simulink library "slexPowerWindowSALib"  (R2014b)
settings: Solver=ode45  SolverMode=SingleTasking  StartTime=0.0  StopTime=10.0  RelTol=1e-3
libraries: slexPowerWindowSALib x4, simulink x2
Description:
  | Library of Components for Control System
settings Model: ExtModeAutoUpdateStatusClock=off  Creator=The MathWorks Inc.  LastModifiedBy=The MathWorks Inc.

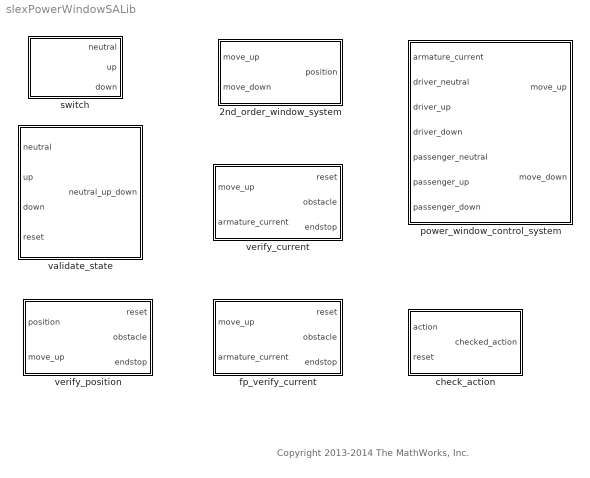
== system slexPowerWindowSALib ==
  note: Copyright 2013-2014 The MathWorks, Inc.
  2nd_order_window_system : Subsystem
  check_action : Subsystem
  fp_verify_current : Subsystem
  power_window_control_system : Subsystem
  switch : Subsystem
  validate_state : Subsystem
  verify_current : Subsystem
  verify_position : Subsystem

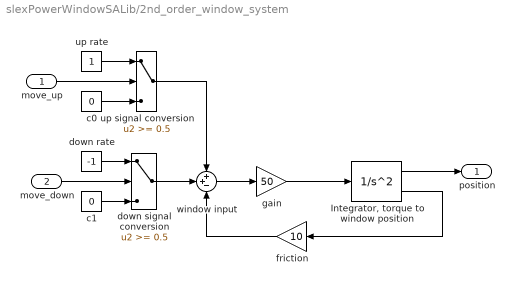
== system slexPowerWindowSALib/2nd_order_window_system ==
  move_up : Inport
  move_down : Inport  Port=2
  "Integrator, torque to window position " : SecondOrderIntegrator
  c0 : Constant  Value=0
  c1 : Constant  Value=0
  down rate : Constant  Value=-1
  down signal conversion : Switch  Threshold=0.5  SaturateOnIntegerOverflow=on  InputSameDT=on
  friction : Gain  Gain=10  SaturateOnIntegerOverflow=on  OutDataTypeStr=Inherit: Same as input  ParamDataTypeStr=Inherit: Same as input
  gain : Gain  Gain=50  SaturateOnIntegerOverflow=on  OutDataTypeStr=Inherit: Same as input  ParamDataTypeStr=Inherit: Same as input
  up rate : Constant
  up signal conversion : Switch  Threshold=0.5  SaturateOnIntegerOverflow=on  InputSameDT=on
  window input : Sum  Inputs=++-  SaturateOnIntegerOverflow=on  InputSameDT=on  OutDataTypeStr=Inherit: Same as first input
  position : Outport
  wires:
  move_down/1 -> down signal conversion/2
  "Integrator, torque to window position "/1 -> position/1
  move_up/1 -> up signal conversion/2
  up rate/1 -> up signal conversion/1
  c0/1 -> up signal conversion/3
  down rate/1 -> down signal conversion/1
  c1/1 -> down signal conversion/3
  up signal conversion/1 -> window input/1
  down signal conversion/1 -> window input/2
  window input/1 -> gain/1
  gain/1 -> "Integrator, torque to window position "/1
  "Integrator, torque to window position "/2 -> friction/1
  friction/1 -> window input/3

== system slexPowerWindowSALib/check_action ==
  action : Inport
  reset : Inport  Port=2
  allow_action : Logic  IconShape=distinctive  OutDataTypeStr=boolean
  overrule : Logic  Operator=NOT  IconShape=distinctive  OutDataTypeStr=boolean
  checked_action : Outport
  wires:
  overrule/1 -> allow_action/2
  action/1 -> allow_action/1
  allow_action/1 -> checked_action/1
  reset/1 -> overrule/1

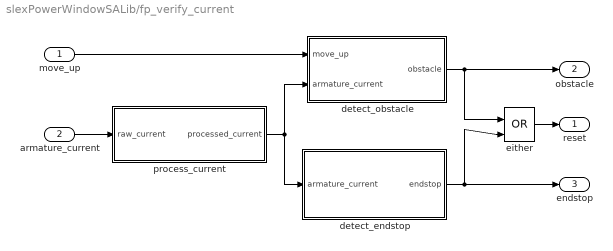
== system slexPowerWindowSALib/fp_verify_current ==
  move_up : Inport  OutDataTypeStr=boolean
  armature_current : Inport  Port=2
  detect_endstop : Subsystem
  detect_obstacle : Subsystem
  either : Logic  Operator=OR  IconShape=distinctive  OutDataTypeStr=boolean
  process_current : Subsystem
  reset : Outport
  obstacle : Outport  Port=2
  endstop : Outport  Port=3
  wires:
  armature_current/1 -> process_current/1(raw_current)
  detect_obstacle/1(obstacle) -> either/1, obstacle/1
  detect_endstop/1(endstop) -> endstop/1, either/2
  either/1 -> reset/1
  move_up/1 -> detect_obstacle/1(move_up)
  process_current/1(processed_current) -> detect_obstacle/2(armature_current), detect_endstop/1(armature_current)

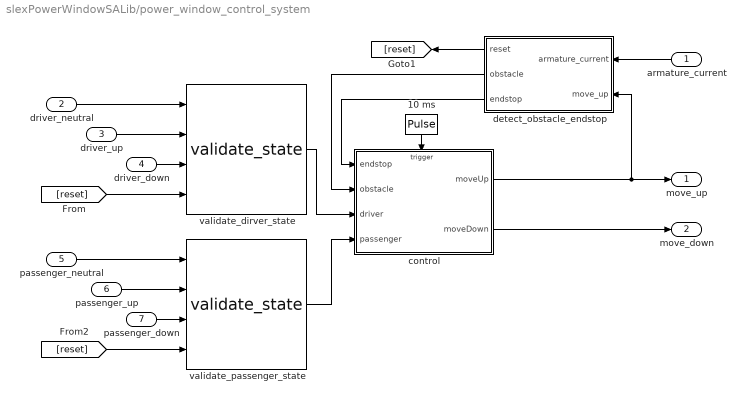
== system slexPowerWindowSALib/power_window_control_system ==
  armature_current : Inport
  driver_neutral : Inport  Port=2
  driver_up : Inport  Port=3
  driver_down : Inport  Port=4
  passenger_neutral : Inport  Port=5
  passenger_up : Inport  Port=6
  passenger_down : Inport  Port=7
  10 ms : DiscretePulseGenerator  PulseType=Time based  Period=1e-2  SampleTime=1e-3
  control : Stateflow chart  TreatAsAtomicUnit=on
  detect_obstacle_endstop : Subsystem
  validate_dirver_state : slexPowerWindowSALib/validate_state
  validate_passenger_state : slexPowerWindowSALib/validate_state
  move_up : Outport
  move_down : Outport  Port=2
  wires:
  armature_current/1 -> detect_obstacle_endstop/1(armature_current)
  control/2(moveDown) -> move_down/1
  control/1(moveUp) -> detect_obstacle_endstop/2(move_up), move_up/1
  detect_obstacle_endstop/3(endstop) -> control/1(endstop)
  detect_obstacle_endstop/2(obstacle) -> control/2(obstacle)
  validate_passenger_state/1 -> control/4(passenger)
  validate_dirver_state/1 -> control/3(driver)
  10 ms/1 -> control/Trigger
  detect_obstacle_endstop/1(reset) -> [reset]
  [reset] -> validate_passenger_state/4
  passenger_down/1 -> validate_passenger_state/3
  passenger_up/1 -> validate_passenger_state/2
  passenger_neutral/1 -> validate_passenger_state/1
  driver_down/1 -> validate_dirver_state/3
  driver_up/1 -> validate_dirver_state/2
  driver_neutral/1 -> validate_dirver_state/1
  [reset] -> validate_dirver_state/4

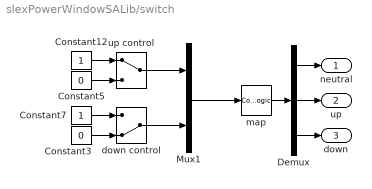
== system slexPowerWindowSALib/switch ==
  Constant12 : Constant  OutDataTypeStr=boolean
  Constant3 : Constant  Value=0  OutDataTypeStr=boolean
  Constant5 : Constant  Value=0  OutDataTypeStr=boolean
  Constant7 : Constant  OutDataTypeStr=boolean
  Demux : Demux  Outputs=3
  Mux1 : Mux  Inputs=2
  down control : ManualSwitch  CurrentSetting=0
  map : CombinatorialLogic  TruthTable=[1 0 0;0 0 1;0 1 0;1 0 0]
  up control : ManualSwitch
  neutral : Outport
  up : Outport  Port=2
  down : Outport  Port=3
  wires:
  Demux/3 -> down/1
  Demux/2 -> up/1
  Demux/1 -> neutral/1
  map/1 -> Demux/1
  up control/1 -> Mux1/1
  down control/1 -> Mux1/2
  Constant3/1 -> down control/2
  Constant7/1 -> down control/1
  Constant5/1 -> up control/2
  Constant12/1 -> up control/1
  Mux1/1 -> map/1

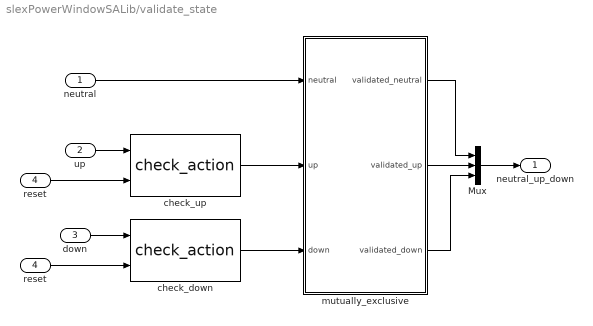
== system slexPowerWindowSALib/validate_state ==
  neutral : Inport
  up : Inport  Port=2
  down : Inport  Port=3
  reset : Inport  Port=4
  Mux : Mux  Inputs=3
  check_down : slexPowerWindowSALib/check_action
  check_up : slexPowerWindowSALib/check_action
  mutually_exclusive : Subsystem
  "reset " : InportShadow  Port=4
  neutral_up_down : Outport
  wires:
  check_down/1 -> mutually_exclusive/3(down)
  mutually_exclusive/3(validated_down) -> Mux/3
  mutually_exclusive/2(validated_up) -> Mux/2
  mutually_exclusive/1(validated_neutral) -> Mux/1
  down/1 -> check_down/1
  up/1 -> check_up/1
  neutral/1 -> mutually_exclusive/1(neutral)
  check_up/1 -> mutually_exclusive/2(up)
  "reset "/1 -> check_up/2
  reset/1 -> check_down/2
  Mux/1 -> neutral_up_down/1

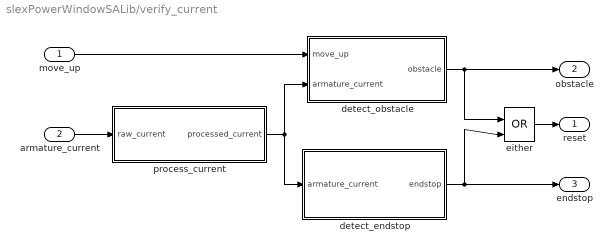
== system slexPowerWindowSALib/verify_current ==
  move_up : Inport  OutDataTypeStr=boolean
  armature_current : Inport  Port=2
  detect_endstop : Subsystem
  detect_obstacle : Subsystem
  either : Logic  Operator=OR  IconShape=distinctive  OutDataTypeStr=boolean
  process_current : Subsystem
  reset : Outport
  obstacle : Outport  Port=2
  endstop : Outport  Port=3
  wires:
  process_current/1(processed_current) -> detect_endstop/1(armature_current), detect_obstacle/2(armature_current)
  move_up/1 -> detect_obstacle/1(move_up)
  either/1 -> reset/1
  detect_endstop/1(endstop) -> either/2, endstop/1
  detect_obstacle/1(obstacle) -> obstacle/1, either/1
  armature_current/1 -> process_current/1(raw_current)

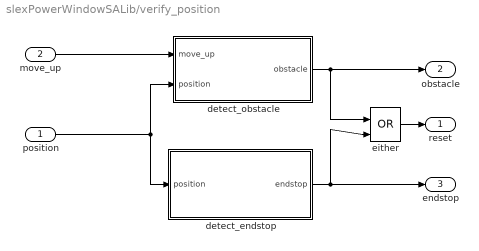
== system slexPowerWindowSALib/verify_position ==
  position : Inport
  move_up : Inport  Port=2  OutDataTypeStr=boolean
  detect_endstop : Subsystem
  detect_obstacle : Subsystem
  either : Logic  Operator=OR  IconShape=distinctive  OutDataTypeStr=boolean
  reset : Outport
  obstacle : Outport  Port=2
  endstop : Outport  Port=3
  wires:
  move_up/1 -> detect_obstacle/1(move_up)
  position/1 -> detect_endstop/1(position), detect_obstacle/2(position)
  either/1 -> reset/1
  detect_endstop/1(endstop) -> either/2, endstop/1
  detect_obstacle/1(obstacle) -> obstacle/1, either/1

== system slexPowerWindowSALib/fp_verify_current/detect_endstop ==
  armature_current : Inport
  current_limit : simulink/Logic and Bit Operations/Compare To Constant  relop=>  const=15  OutDataTypeStr=boolean
  endstop : Outport
  wires:
  current_limit/1 -> endstop/1
  armature_current/1 -> current_limit/1

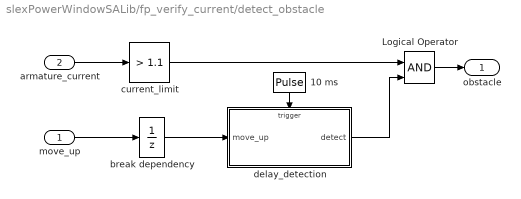
== system slexPowerWindowSALib/fp_verify_current/detect_obstacle ==
  move_up : Inport  OutDataTypeStr=boolean
  armature_current : Inport  Port=2
  10 ms : DiscretePulseGenerator  SampleTime=10e-3
  Logical Operator : Logic  IconShape=distinctive  AllPortsSameDT=off  OutDataTypeStr=boolean
  break dependency : UnitDelay  SampleTime=0.01
  current_limit : simulink/Logic and Bit Operations/Compare To Constant  relop=>  const=1.1  OutDataTypeStr=boolean
  delay_detection : Stateflow chart  TreatAsAtomicUnit=on
  obstacle : Outport
  wires:
  break dependency/1 -> delay_detection/1(move_up)
  10 ms/1 -> delay_detection/Trigger
  move_up/1 -> break dependency/1
  armature_current/1 -> current_limit/1
  delay_detection/1(" detect") -> Logical Operator/2
  current_limit/1 -> Logical Operator/1
  Logical Operator/1 -> obstacle/1

== system slexPowerWindowSALib/fp_verify_current/process_current ==
  raw_current : Inport
  3.5 / (2^(bits-1)) : Gain  Gain=0.02734375  OutDataTypeStr=fixdt(1,16,6)
  Abs : Abs
  gain : Gain  Gain=5  OutDataTypeStr=fixdt(1,16,5)
  processed_current : Outport
  wires:
  raw_current/1 -> 3.5 / (2^(bits-1))/1
  Abs/1 -> processed_current/1
  gain/1 -> Abs/1
  3.5 / (2^(bits-1))/1 -> gain/1

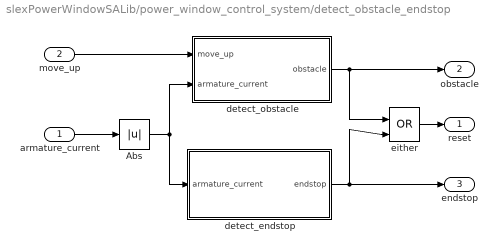
== system slexPowerWindowSALib/power_window_control_system/detect_obstacle_endstop ==
  armature_current : Inport
  move_up : Inport  Port=2
  Abs : Abs  SaturateOnIntegerOverflow=on
  detect_endstop : Subsystem
  detect_obstacle : Subsystem
  either : Logic  Operator=OR  IconShape=distinctive  OutDataTypeStr=boolean
  reset : Outport
  obstacle : Outport  Port=2
  endstop : Outport  Port=3
  wires:
  detect_obstacle/1(obstacle) -> either/1, obstacle/1
  detect_endstop/1(endstop) -> endstop/1, either/2
  either/1 -> reset/1
  armature_current/1 -> Abs/1
  move_up/1 -> detect_obstacle/1(move_up)
  Abs/1 -> detect_endstop/1(armature_current), detect_obstacle/2(armature_current)

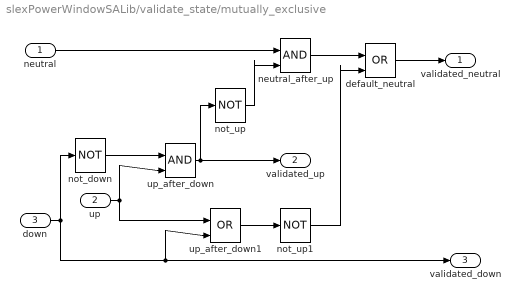
== system slexPowerWindowSALib/validate_state/mutually_exclusive ==
  neutral : Inport
  up : Inport  Port=2
  down : Inport  Port=3
  default_neutral : Logic  Operator=OR  IconShape=distinctive  OutDataTypeStr=boolean
  neutral_after_up : Logic  IconShape=distinctive  OutDataTypeStr=boolean
  not_down : Logic  Operator=NOT  IconShape=distinctive  OutDataTypeStr=boolean
  not_up : Logic  Operator=NOT  IconShape=distinctive  OutDataTypeStr=boolean
  not_up1 : Logic  Operator=NOT  IconShape=distinctive  OutDataTypeStr=boolean
  up_after_down : Logic  IconShape=distinctive  OutDataTypeStr=boolean
  up_after_down1 : Logic  Operator=OR  IconShape=distinctive  OutDataTypeStr=boolean
  validated_neutral : Outport
  validated_up : Outport  Port=2
  validated_down : Outport  Port=3
  wires:
  not_up1/1 -> default_neutral/2
  default_neutral/1 -> validated_neutral/1
  neutral_after_up/1 -> default_neutral/1
  up_after_down1/1 -> not_up1/1
  up/1 -> up_after_down/2, up_after_down1/1
  neutral/1 -> neutral_after_up/1
  down/1 -> validated_down/1, up_after_down1/2, not_down/1
  not_up/1 -> neutral_after_up/2
  up_after_down/1 -> validated_up/1, not_up/1
  not_down/1 -> up_after_down/1

== system slexPowerWindowSALib/verify_current/detect_endstop ==
  armature_current : Inport
  Constant6 : Constant  Value=15
  current_limit : RelationalOperator  Operator=>  OutDataTypeStr=boolean  InputSameDT=on
  endstop : Outport
  wires:
  Constant6/1 -> current_limit/2
  armature_current/1 -> current_limit/1
  current_limit/1 -> endstop/1

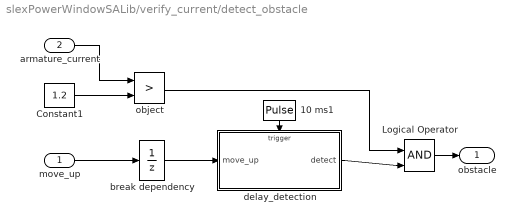
== system slexPowerWindowSALib/verify_current/detect_obstacle ==
  move_up : Inport  OutDataTypeStr=boolean
  armature_current : Inport  Port=2
  10 ms1 : DiscretePulseGenerator  SampleTime=10e-3
  Constant1 : Constant  Value=1.2
  Logical Operator : Logic  IconShape=distinctive  AllPortsSameDT=off  OutDataTypeStr=boolean
  break dependency : UnitDelay  SampleTime=0.01
  delay_detection : Stateflow chart  TreatAsAtomicUnit=on
  object : RelationalOperator  Operator=>  OutDataTypeStr=boolean  InputSameDT=on
  obstacle : Outport
  wires:
  Constant1/1 -> object/2
  object/1 -> Logical Operator/1
  delay_detection/1(" detect") -> Logical Operator/2
  armature_current/1 -> object/1
  move_up/1 -> break dependency/1
  10 ms1/1 -> delay_detection/Trigger
  break dependency/1 -> delay_detection/1(move_up)
  Logical Operator/1 -> obstacle/1

== system slexPowerWindowSALib/verify_current/process_current ==
  raw_current : Inport
  Abs : Abs  SaturateOnIntegerOverflow=on
  processed_current : Outport
  wires:
  Abs/1 -> processed_current/1
  raw_current/1 -> Abs/1

== system slexPowerWindowSALib/verify_position/detect_endstop ==
  position : Inport
  Constant1 : Constant  Value=0
  Constant6 : Constant  Value=0.4
  Logical Operator : Logic  Operator=OR  IconShape=distinctive  AllPortsSameDT=off  OutDataTypeStr=boolean
  bottom_limit : RelationalOperator  Operator=<  OutDataTypeStr=boolean  InputSameDT=on
  top_limit : RelationalOperator  Operator=>  OutDataTypeStr=boolean  InputSameDT=on
  endstop : Outport
  wires:
  Constant6/1 -> top_limit/2
  position/1 -> bottom_limit/1, top_limit/1
  Constant1/1 -> bottom_limit/2
  top_limit/1 -> Logical Operator/1
  bottom_limit/1 -> Logical Operator/2
  Logical Operator/1 -> endstop/1

== system slexPowerWindowSALib/verify_position/detect_obstacle ==
  move_up : Inport  OutDataTypeStr=boolean
  position : Inport  Port=2
  Break Dependency : Memory
  Constant1 : Constant  Value=0.3
  Logical Operator : Logic  IconShape=distinctive  AllPortsSameDT=off  OutDataTypeStr=boolean
  object : RelationalOperator  Operator=>  OutDataTypeStr=boolean  InputSameDT=on
  obstacle : Outport
  wires:
  Constant1/1 -> object/2
  object/1 -> Logical Operator/1
  position/1 -> object/1
  move_up/1 -> Break Dependency/1
  Break Dependency/1 -> Logical Operator/2
  Logical Operator/1 -> obstacle/1

== system slexPowerWindowSALib/power_window_control_system/detect_obstacle_endstop/detect_endstop ==
  armature_current : Inport
  Constant6 : Constant  Value=15
  current_limit : RelationalOperator  Operator=>  OutDataTypeStr=boolean  InputSameDT=on
  endstop : Outport
  wires:
  current_limit/1 -> endstop/1
  armature_current/1 -> current_limit/1
  Constant6/1 -> current_limit/2

== system slexPowerWindowSALib/power_window_control_system/detect_obstacle_endstop/detect_obstacle ==
  move_up : Inport
  armature_current : Inport  Port=2
  Constant1 : Constant  Value=1.6
  Logical Operator : Logic  IconShape=distinctive  AllPortsSameDT=off  OutDataTypeStr=boolean
  break dependency : UnitDelay  SampleTime=0.01
  delay 500 ms : Subsystem  TreatAsAtomicUnit=on
  object : RelationalOperator  Operator=>  OutDataTypeStr=boolean  InputSameDT=on
  obstacle : Outport
  wires:
  break dependency/1 -> delay 500 ms/Enable
  Logical Operator/1 -> obstacle/1
  move_up/1 -> break dependency/1
  armature_current/1 -> object/1
  delay 500 ms/1(step) -> Logical Operator/2
  object/1 -> Logical Operator/1
  Constant1/1 -> object/2

== system slexPowerWindowSALib/power_window_control_system/detect_obstacle_endstop/detect_obstacle/delay 500 ms ==
  Enable : EnablePort  StatesWhenEnabling=reset
  Constant : Constant
  Constant1 : Constant  Value=0.5
  Integrator : Integrator
  Relational Operator : RelationalOperator  Operator=>  OutDataTypeStr=boolean  InputSameDT=on
  step : Outport  OutputWhenDisabled=reset  InitialOutput=0
  wires:
  Relational Operator/1 -> step/1
  Constant1/1 -> Relational Operator/2
  Integrator/1 -> Relational Operator/1
  Constant/1 -> Integrator/1

== stateflow chart slexPowerWindowSALib/power_window_control_system/control ==
  settings: executeAtInitialization=1
  state safe
    state driverNeutral
      entry:
      moveUp = 0;
      moveDown = 0;
      state passengerneutral
        entry:
        moveUp = 0;
        moveDown = 0;
      state passengerDown
        entry: moveDown = 1;
        exit: moveDown = 0;
        state iniPassengerDown
        state passengerDown
        state autoPassengerDown
        iniPassengerDown -> (junction 54) : after(100,ticks)
        (junction 54) -> autoPassengerDown [order 1] : [passenger[1]]
        (junction 54) -> safe.driverNeutral.passengerDown.passengerDown [order 2]
      state passengerUp
        entry: moveUp = 1;
        exit: moveUp = 0;
        state iniPassengerUp
        state PassengerUp
        state autoPassengerUp
        iniPassengerUp -> (junction 55) : after(100,ticks)
        (junction 55) -> PassengerUp [order 2]
        (junction 55) -> autoPassengerUp [order 1] : [passenger[1]]
      (default) -> passengerneutral
      passengerneutral -> iniPassengerUp [order 1] : [passenger[2]]
      passengerneutral -> iniPassengerDown [order 2] : [passenger[3]]
      safe.driverNeutral.passengerDown.passengerDown -> passengerneutral : [passenger[1]]
      safe.driverNeutral.passengerDown -> passengerneutral [order 1] : [endstop]
      PassengerUp -> passengerneutral : [passenger[1]]
      passengerUp -> passengerneutral [order 2] : [endstop]
      safe.driverNeutral.passengerDown -> PassengerUp [order 2] : [passenger[2]]
      passengerUp -> safe.driverNeutral.passengerDown.passengerDown [order 1] : [passenger[3]]
    state driverDown
      entry: moveDown = 1;
      exit: moveDown = 0;
      state iniDriverDown
      state autoDriverDown
      state DriverDown
      iniDriverDown -> (junction 56) : after(100,ticks)
      (junction 56) -> autoDriverDown [order 1] : [driver[1]]
      (junction 56) -> DriverDown [order 2]
    state driverUp
      entry: moveUp = 1;
      exit: moveUp = 0;
      state iniDriverUp
      state DriverUp
      state autoDriverUp
      iniDriverUp -> (junction 57) : after(100,ticks)
      (junction 57) -> DriverUp [order 2]
      (junction 57) -> autoDriverUp [order 1] : [driver[1]]
    (default) -> driverNeutral
    driverNeutral -> iniDriverDown [order 2] : [driver[3]]
    DriverDown -> driverNeutral : [driver[1]]
    driverDown -> driverNeutral [order 1] : [endstop]
    DriverUp -> driverNeutral : [driver[1]]
    driverUp -> driverNeutral [order 2] : [endstop]
    driverNeutral -> iniDriverUp [order 1] : [driver[2]]
    driverDown -> DriverUp [order 2] : [driver[2]]
    driverUp -> DriverDown [order 1] : [driver[3]]
  state emergencyDown
    entry:
    moveUp = 0;
    moveDown = 1;
  emergencyDown -> passengerneutral : [endstop | after(100,ticks)]
  (default) -> safe
  safe -> emergencyDown : [obstacle]
  data: moveUp output boolean; moveDown output boolean; endstop input boolean; obstacle input boolean; driver input boolean size=3; passenger input boolean size=3
  events: ticks input RISING_EDGE_EVENT

== stateflow chart slexPowerWindowSALib/verify_current/detect_obstacle/delay_detection ==
  settings: executeAtInitialization=1
  state off
  state hold
  state detect
  (default) -> off
  off -> hold : [move_up]
  detect -> off : [~move_up]
  hold -> off [order 2] : [~move_up]
  hold -> detect [order 1] : [after(100,ticks)]
  data: detect output unknown; move_up input boolean
  events: ticks input EITHER_EDGE_EVENT

== stateflow chart slexPowerWindowSALib/fp_verify_current/detect_obstacle/delay_detection ==
  settings: executeAtInitialization=1
  state off
  state hold
  state detect
  (default) -> off
  off -> hold : [move_up]
  detect -> off : [~move_up]
  hold -> off [order 2] : [~move_up]
  hold -> detect [order 1] : [after(100,ticks)]
  data: detect output unknown; move_up input boolean
  events: ticks input EITHER_EDGE_EVENT
